simulink subsystem "H3LIS331DLTR"  (R2025b)
settings: Solver=VariableStepAuto  StartTime=0.0  StopTime=10.0  RelTol=1e-3
undefined symbols (not defined in the file): ba_high_init
settings Model: Creator=jak64  LastModifiedBy=slee7

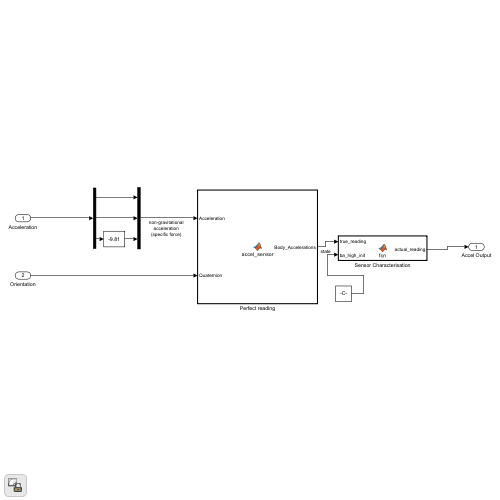
[thumbnail: Simulink's stored preview of the top-level diagram]
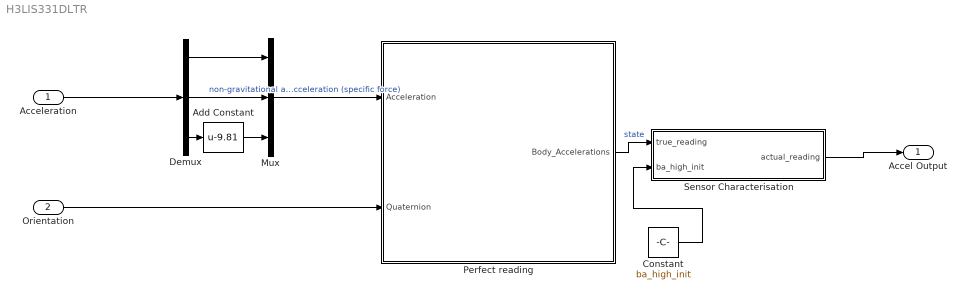
== system H3LIS331DLTR ==
  Acceleration : Inport
  Orientation : Inport  Port=2
  Add Constant : Bias  Bias=-9.81  SaturateOnIntegerOverflow=off
  Constant : Constant  Value=ba_high_init
  Demux : Demux  Outputs=3
  Mux : Mux  Inputs=3
  Perfect reading : MATLAB Function  TreatAsAtomicUnit=on
  Sensor Characterisation : MATLAB Function  TreatAsAtomicUnit=on
  Accel Output : Outport
  wires:
  Acceleration/1 -> Demux/1
  Orientation/1 -> Perfect reading/2(Quaternion)
  Demux/3 -> Add Constant/1
  Mux/1 -> Perfect reading/1(Acceleration)  "non-gravitational acceleration (specific force)"
  Demux/2 -> Mux/2
  Demux/1 -> Mux/1
  Add Constant/1 -> Mux/3
  Sensor Characterisation/1(actual_reading) -> Accel Output/1
  Perfect reading/1(Body_Accelerations) -> Sensor Characterisation/1(true_reading)  "state"
  Constant/1 -> Sensor Characterisation/2(ba_high_init)

== matlab function H3LIS331DLTR/Perfect reading ==
  data: Acceleration input; Body_Accelerations output; Quaternion input
function Body_Accelerations = accel_sensor(Acceleration, Quaternion)
%#codegen
Body_Accelerations = ned2body(Acceleration, Quaternion);
end

== matlab function H3LIS331DLTR/Sensor Characterisation ==
  data: true_reading input; actual_reading output; ba_high_init input
function actual_reading = fcn(true_reading, ba_high_init)
    persistent b_previous

    dt = 0.0553; % Simulation Time Step[s]

    % Bias: Composite Bias = Const + Gauss-Markov Drift
    
        b_const = ba_high_init'; % Constant bias
    
        % Drift bias (b = exp^-dt/tau * b_previous + omega)
        
        if isempty(b_previous)
            b_previous = [0; 0; 0]; 
        end
    
        tau = [8.731; 8.731; 8.731]; % time constant of drift
        q = [8.774166e-04; 7.720775e-04; 1.336849e-03]; % variance on drift
    
        omega = sqrt(q) .* randn(3,1); % omega ~ N(0,q)
        
        b_drift = exp(-dt ./ tau) .* b_previous + omega;
    
        composite_bias = b_const + b_drift; 

    % Noise: Gaussian  

        noise_variance = [1.645664; 1.487596; 1.836378]; 
    
        noise = noise_variance .* randn(3,1); 
    
    % Quantisation:

        quant_step = 0.5; % Quant Step: data sheet
   

    % Reading Processing:

        actual_reading_continuous  = true_reading(:) + composite_bias + noise;

        actual_reading_quantised = quant_step .* round(actual_reading_continuous ./ quant_step);

        actual_reading = actual_reading_quantised; 

end

% Currently Ignoring: 
% Scale_factor_error 
% Misalignment_error
